simulink model "model_3"  (R2014a)
settings: Solver=ode3  StartTime=0.0  StopTime=30  FixedStep=0.1  RelTol=1e-3
settings Model: Creator=Павел  LastModifiedBy=Павел

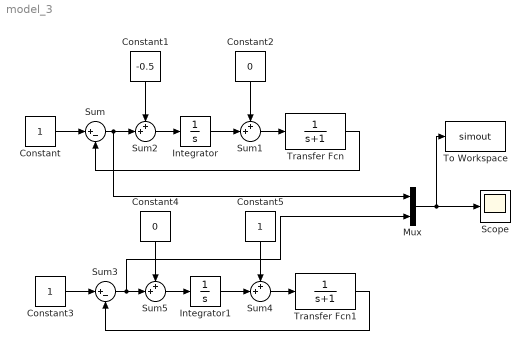
== system model_3 ==
  Constant : Constant
  Constant1 : Constant  Value=-0.5
  Constant2 : Constant  Value=0
  Constant3 : Constant
  Constant4 : Constant  Value=0
  Constant5 : Constant
  Integrator : Integrator
  Integrator1 : Integrator
  Mux : Mux  Inputs=2
  Scope : Scope
  Sum : Sum  Inputs=|+-
  Sum{1..2,4..5} (4 alike) : Sum  Inputs=++|
  Sum3 : Sum  Inputs=|+-
  To Workspace : ToWorkspace  VariableName=simout  SaveFormat=Structure With Time  SampleTime=-1
  Transfer Fcn : TransferFcn  Denominator=[1 1]
  Transfer Fcn1 : TransferFcn  Denominator=[1 1]
  wires:
  Sum1/1 -> Transfer Fcn/1
  Integrator/1 -> Sum1/2
  Sum2/1 -> Integrator/1
  Sum/1 -> Mux/1, Sum2/2
  Constant/1 -> Sum/1
  Transfer Fcn/1 -> Sum/2
  Constant1/1 -> Sum2/1
  Constant2/1 -> Sum1/1
  Sum4/1 -> Transfer Fcn1/1
  Integrator1/1 -> Sum4/2
  Sum5/1 -> Integrator1/1
  Sum3/1 -> Mux/2, Sum5/2
  Constant3/1 -> Sum3/1
  Transfer Fcn1/1 -> Sum3/2
  Constant4/1 -> Sum5/1
  Constant5/1 -> Sum4/1
  Mux/1 -> To Workspace/1, Scope/1
